simulink model "flightControlSystem"  (R2020a)
settings: Solver=ode3  StartTime=0  StopTime=TFinal  FixedStep=Ts  RelTol=1e-3  EnableMultiTasking=on
undefined symbols (not defined in the file): codertarget, Controller, DiscIntNeverNeededParam, Discrete, Estimator, g, gray, init, orient_ref, pos_ref, Sensors, Time, Ts, Vehicle
libraries: simulink x35, sharedtransform x3, ctrlSharedLib x2, sharedutil x1, visionstatistics x1, simulink_extras x1, parrotlib x1
(part 2 of 2)

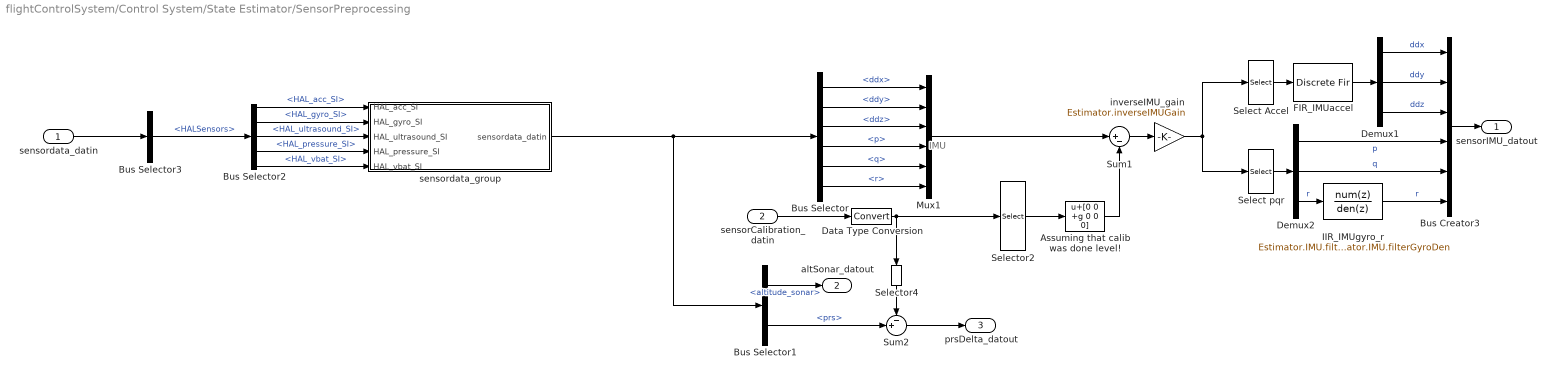
== system flightControlSystem/Control System/State Estimator/SensorPreprocessing ==
  note: IMU
  sensordata_datin : Inport
  sensorCalibration_datin : Inport  Port=2
  Assuming that calib was done level! : Bias  Bias=[0 0 +g 0 0 0]
  Bus Creator3 : BusCreator  Inputs=6
  Bus Selector : BusSelector  OutputSignals=ddx,ddy,ddz,p,q,r
  Bus Selector1 : BusSelector  OutputSignals=altitude_sonar,prs
  Bus Selector2 : BusSelector  OutputSignals=HAL_acc_SI,HAL_gyro_SI,HAL_ultrasound_SI,HAL_pressure_SI,HAL_vbat_SI
  Bus Selector3 : BusSelector  OutputSignals=HALSensors
  Data Type Conversion : DataTypeConversion
  Demux1 : Demux  Outputs=3
  Demux2 : Demux  Outputs=3
  FIR_IMUaccel : DiscreteFir  Coefficients=Estimator.IMU.filterAccel.Coefficients
  IIR_IMUgyro_r : DiscreteFilter  Numerator=Estimator.IMU.filterGyroNum  Denominator=Estimator.IMU.filterGyroDen
  Mux1 : Mux  Inputs=6
  Select Accel : Selector  InputPortWidth=6  IndexOptions=Index vector (dialog)  Indices=[1 2 3]  OutputSizes=1
  Select pqr : Selector  InputPortWidth=6  IndexOptions=Index vector (dialog)  Indices=[4 5 6]  OutputSizes=1
  Selector2 : Selector  InputPortWidth=8  IndexOptions=Index vector (dialog)  Indices=[1:6]  OutputSizes=1
  Selector4 : Selector  InputPortWidth=8  IndexOptions=Index vector (dialog)  Indices=[7]  OutputSizes=1
  Sum1 : Sum  Inputs=|+-
  Sum2 : Sum  Inputs=-+|
  inverseIMU_gain : Gain  Gain=Estimator.inverseIMUGain  ParamDataTypeStr=single  OutDataTypeStr=single
  sensordata_group : Subsystem
  sensorIMU_datout : Outport  VectorParamsAs1DForOutWhenUnconnected=off
  altSonar_datout : Outport  Port=2  VectorParamsAs1DForOutWhenUnconnected=off
  prsDelta_datout : Outport  Port=3  VectorParamsAs1DForOutWhenUnconnected=off
  wires:
  Select pqr/1 -> Demux2/1
  Assuming that calib was done level!/1 -> Sum1/2
  Mux1/1 -> Sum1/1
  Sum2/1 -> prsDelta_datout/1
  Bus Selector1/2 -> Sum2/2  "<prs>"
  Selector4/1 -> Sum2/1
  Bus Selector1/1 -> altSonar_datout/1  "<altitude_sonar>"
  Bus Selector/6 -> Mux1/6  "<r>"
  Bus Selector/5 -> Mux1/5  "<q>"
  Bus Selector/4 -> Mux1/4  "<p>"
  Bus Selector/3 -> Mux1/3  "<ddz>"
  Bus Selector/2 -> Mux1/2  "<ddy>"
  Bus Selector/1 -> Mux1/1  "<ddx>"
  sensorCalibration_datin/1 -> Data Type Conversion/1
  IIR_IMUgyro_r/1 -> Bus Creator3/6  "r"
  Demux2/3 -> IIR_IMUgyro_r/1  "r"
  FIR_IMUaccel/1 -> Demux1/1
  Select Accel/1 -> FIR_IMUaccel/1
  inverseIMU_gain/1 -> Select Accel/1, Select pqr/1
  Demux2/2 -> Bus Creator3/5  "q"
  Demux2/1 -> Bus Creator3/4  "p"
  Selector2/1 -> Assuming that calib was done level!/1
  Sum1/1 -> inverseIMU_gain/1
  Demux1/3 -> Bus Creator3/3  "ddz"
  Demux1/2 -> Bus Creator3/2  "ddy"
  Demux1/1 -> Bus Creator3/1  "ddx"
  Bus Creator3/1 -> sensorIMU_datout/1
  Data Type Conversion/1 -> Selector2/1, Selector4/1
  Bus Selector2/2 -> sensordata_group/2(HAL_gyro_SI)  "<HAL_gyro_SI>"
  Bus Selector2/4 -> sensordata_group/4(HAL_pressure_SI)  "<HAL_pressure_SI>"
  Bus Selector2/5 -> sensordata_group/5(HAL_vbat_SI)  "<HAL_vbat_SI>"
  Bus Selector2/3 -> sensordata_group/3(HAL_ultrasound_SI)  "<HAL_ultrasound_SI>"
  Bus Selector3/1 -> Bus Selector2/1  "<HALSensors>"
  sensordata_group/1(sensordata_datin) -> Bus Selector1/1, Bus Selector/1
  sensordata_datin/1 -> Bus Selector3/1
  Bus Selector2/1 -> sensordata_group/1(HAL_acc_SI)  "<HAL_acc_SI>"

== system flightControlSystem/Control System/Path Planning1/take current yaw, x and y targets in pixels, output the target orientation/create scaled x and y coordinates for finding an error angle less prone to fluctuation ==
  phi : Inport
  " y component in arbitrary coordinates" : Trigonometry
  scale y to reduce the angle : Gain  Gain=6
  x component in arbitrary coordinates : Trigonometry  Operator=cos
  x : Outport
  y : Outport  Port=2
  wires:
  phi/1 -> x component in arbitrary coordinates/1, " y component in arbitrary coordinates"/1
  scale y to reduce the angle/1 -> y/1
  " y component in arbitrary coordinates"/1 -> scale y to reduce the angle/1
  x component in arbitrary coordinates/1 -> x/1

== system flightControlSystem/Control System/Path Planning1/take current yaw, x and y targets in pixels, output the target orientation/output the desired yaw ==
  note: Subsystem
  note: Find the difference between absolute and relative angle
  note: relative angle, correction for 0 degrees at north (instead of east)
  note: Pump this through a logistic function so that smaller relative theta values are scaled less
  <yaw> : Inport
  a : Inport  Port=2
  Chart : Stateflow chart  TreatAsAtomicUnit=on
  Constant : Constant  Value=0
  Constant1 : Constant  Value=0
  Constant4 : Constant  Value=pi/2
  MATLAB Function : MATLAB Function  TreatAsAtomicUnit=on
  Minus2 : Sum  Inputs=+-
  Minus3 : Sum
  Scope : Scope
  z : Outport
  Out2 : Outport  Port=2
  Out3 : Outport  Port=3
  wires:
  Constant1/1 -> Out3/1
  Chart/1(z) -> z/1, Scope/1
  Minus3/1 -> Chart/1(input_theta)
  Constant4/1 -> Minus2/1
  Constant/1 -> Out2/1
  MATLAB Function/1(y) -> Minus3/2
  Minus2/1 -> MATLAB Function/1(u)
  a/1 -> Minus2/2
  <yaw>/1 -> Minus3/1

== system flightControlSystem/Control System/Path Planning1/take current yaw, x and y targets in pixels, output the target orientation/relative angle Phi of the pixel centre to the centre of mass measured anticlockwise from east in the frame of the drone ==
  note: angle in frame 1
  note: delX
  note: delY
  xcom : Inport
  ycom : Inport  Port=2
  Atan2 : Trigonometry  Operator=atan2
  Minus : Sum  Inputs=+-
  Minus1 : Sum  Inputs=+-
  x_pixel_grid_centre : Constant  Value=80
  y_pixel_grid_centre : Constant  Value=60
  Phi : Outport
  wires:
  xcom/1 -> Minus1/1
  y_pixel_grid_centre/1 -> Minus/1
  ycom/1 -> Minus/2
  Minus1/1 -> Atan2/2
  Minus/1 -> Atan2/1
  x_pixel_grid_centre/1 -> Minus1/2
  Atan2/1 -> Phi/1

== system flightControlSystem/Control System/Path Planning1/take current yaw, x and y targets in pixels, output the target orientation1/create scaled x and y coordinates for finding an error angle less prone to fluctuation ==
  phi : Inport
  " y component in arbitrary coordinates" : Trigonometry
  scale y to reduce the angle : Gain  Gain=2
  x component in arbitrary coordinates : Trigonometry  Operator=cos
  x : Outport
  y : Outport  Port=2
  wires:
  phi/1 -> x component in arbitrary coordinates/1, " y component in arbitrary coordinates"/1
  scale y to reduce the angle/1 -> y/1
  " y component in arbitrary coordinates"/1 -> scale y to reduce the angle/1
  x component in arbitrary coordinates/1 -> x/1

== system flightControlSystem/Control System/Path Planning1/take current yaw, x and y targets in pixels, output the target orientation1/output the desired yaw ==
  note: Subsystem
  note: Find the difference between absolute and relative angle
  note: relative angle, correction for 0 degrees at north (instead of east)
  note: Pump this through a logistic function so that smaller relative theta values are scaled less
  <yaw> : Inport
  a : Inport  Port=2
  Chart : Stateflow chart  TreatAsAtomicUnit=on
  Constant : Constant  Value=0
  Constant1 : Constant  Value=0
  Constant4 : Constant  Value=pi/2
  MATLAB Function : MATLAB Function  TreatAsAtomicUnit=on
  Minus2 : Sum  Inputs=+-
  Minus3 : Sum
  Scope : Scope
  z : Outport
  Out2 : Outport  Port=2
  Out3 : Outport  Port=3
  wires:
  Constant1/1 -> Out3/1
  Chart/1(z) -> z/1, Scope/1
  Minus3/1 -> Chart/1(input_theta)
  Constant4/1 -> Minus2/1
  Constant/1 -> Out2/1
  MATLAB Function/1(y) -> Minus3/2
  Minus2/1 -> MATLAB Function/1(u)
  a/1 -> Minus2/2
  <yaw>/1 -> Minus3/1

== system flightControlSystem/Control System/Path Planning1/take current yaw, x and y targets in pixels, output the target orientation1/relative angle Phi of the pixel centre to the centre of mass measured anticlockwise from east in the frame of the drone ==
  note: angle in frame 1
  note: delX
  note: delY
  xcom : Inport
  ycom : Inport  Port=2
  Atan2 : Trigonometry  Operator=atan2
  Minus : Sum  Inputs=+-
  Minus1 : Sum  Inputs=+-
  x_pixel_grid_centre : Constant  Value=80
  y_pixel_grid_centre : Constant  Value=60
  Phi : Outport
  wires:
  xcom/1 -> Minus1/1
  y_pixel_grid_centre/1 -> Minus/1
  ycom/1 -> Minus/2
  Minus1/1 -> Atan2/2
  Minus/1 -> Atan2/1
  x_pixel_grid_centre/1 -> Minus1/2
  Atan2/1 -> Phi/1

== system flightControlSystem/Control System/State Estimator/Complementary Filter/If Action Subsystem ==
  rpy : Inport
  accel : Inport  Port=2
  Action Port : ActionPort  ActionPortLabel=if(u1 > 0)
  Demux : Demux  Outputs=3
  Demux1 : Demux  Outputs=3
  Divide : Product  Inputs=*/
  Gain : Gain  Gain=1-Estimator.gyroAngleUpdateAccWeight
  Gain1 : Gain  Gain=Estimator.gyroAngleUpdateAccWeight
  Gain2 : Gain  Gain=1/g
  Gain3 : Gain  Gain=Estimator.gyroAngleUpdateAccWeight
  Gain4 : Gain  Gain=1-Estimator.gyroAngleUpdateAccWeight
  Mux : Mux  Inputs=2
  Sum : Sum  Inputs=|++
  Sum1 : Sum  Inputs=|++
  Terminator1 : Terminator
  Trigonometric Function : Trigonometry  Operator=atan
  Trigonometric Function1 : Trigonometry  Operator=asin
  pitch,roll : Outport  VectorParamsAs1DForOutWhenUnconnected=off
  wires:
  accel/1 -> Demux/1
  Demux/2 -> Divide/1
  Demux/3 -> Divide/2
  Divide/1 -> Trigonometric Function/1
  Gain/1 -> Sum/1
  Trigonometric Function/1 -> Gain1/1
  Mux/1 -> pitch,roll/1
  Gain2/1 -> Trigonometric Function1/1
  Trigonometric Function1/1 -> Gain3/1
  Gain4/1 -> Sum1/1
  Gain3/1 -> Sum1/2
  Sum1/1 -> Mux/1
  Sum/1 -> Mux/2
  rpy/1 -> Demux1/1
  Demux1/1 -> Gain/1
  Demux1/2 -> Gain4/1
  Demux/1 -> Gain2/1
  Demux1/3 -> Terminator1/1
  Gain1/1 -> Sum/2

== system flightControlSystem/Control System/State Estimator/Complementary Filter/If Action Subsystem2 ==
  prin : Inport
  Action Port : ActionPort  ActionPortLabel=else
  prout : Outport  VectorParamsAs1DForOutWhenUnconnected=off
  wires:
  prin/1 -> prout/1

== system flightControlSystem/Control System/State Estimator/Complementary Filter/Wbe ==
  rpy : Inport  OutDataTypeStr=single
  Constant : Constant  Value=single(0)
  Create 3x3 Matrix : sharedutil/Create 3x3 Matrix  aMode=aMode
      settings: SourceProductBaseCode=AE,PW,MT,VE,VP
  Divide : Product  Inputs=*/
  Gain : Gain  Gain=-1
  Product{1..4} (4 alike) : Product
  Selector : Selector  InputPortWidth=3  IndexOptions=Index vector (dialog)  Indices=[1]  OutputSizes=1
  Selector1 : Selector  InputPortWidth=3  IndexOptions=Index vector (dialog)  Indices=[1]  OutputSizes=1
  Selector2 : Selector  InputPortWidth=3  IndexOptions=Index vector (dialog)  Indices=[2]  OutputSizes=1
  Selector3 : Selector  InputPortWidth=3  IndexOptions=Index vector (dialog)  Indices=[2]  OutputSizes=1
  Trigonometric Function : Trigonometry  Operator=sincos
  Wbe : Outport  VectorParamsAs1DForOutWhenUnconnected=off
  wires:
  Create 3x3 Matrix/1 -> Divide/1
  Product3/1 -> Create 3x3 Matrix/8
  Trigonometric Function/2 -> Selector1/1, Selector2/1
  Selector3/1 -> Product4/2, Product3/2
  Selector1/1 -> Product4/1, Product1/1, Create 3x3 Matrix/3
  Trigonometric Function/1 -> Selector3/1, Selector/1
  Product1/1 -> Create 3x3 Matrix/5
  Product2/1 -> Create 3x3 Matrix/6
  Selector2/1 -> Divide/2, Create 3x3 Matrix/7, Product2/1, Product1/2
  Gain/1 -> Product2/2
  Product4/1 -> Create 3x3 Matrix/9
  Constant/1 -> Create 3x3 Matrix/4, Create 3x3 Matrix/1
  Divide/1 -> Wbe/1
  rpy/1 -> Trigonometric Function/1
  Selector/1 -> Product3/1, Gain/1, Create 3x3 Matrix/2

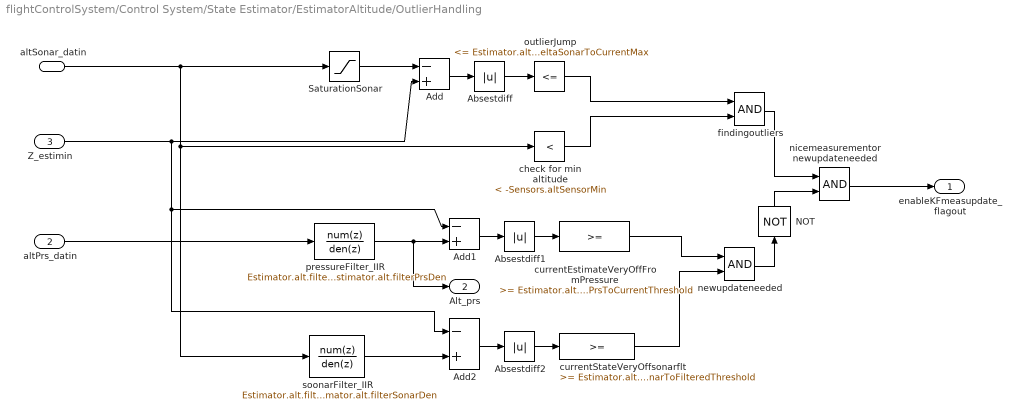
== system flightControlSystem/Control System/State Estimator/EstimatorAltitude/OutlierHandling ==
  altSonar_datin : Inport
  altPrs_datin : Inport  Port=2
  Z_estimin : Inport  Port=3
  Absestdiff : Abs
  Absestdiff1 : Abs
  Absestdiff2 : Abs
  Add : Sum  Inputs=-+
  Add1 : Sum  Inputs=-+
  Add2 : Sum  Inputs=-+
  NOT : Logic  Operator=NOT  IconShape=distinctive  AllPortsSameDT=off  OutDataTypeStr=boolean
  SaturationSonar : Saturate  UpperLimit=-Sensors.altSensorMin  LowerLimit=-inf
  check for min altitude : simulink/Logic and Bit Operations/Compare To Constant  relop=<  const=-Sensors.altSensorMin  OutDataTypeStr=boolean
  currentEstimateVeryOffFromPressure : simulink/Logic and Bit Operations/Compare To Constant  relop=>=  const=Estimator.alt.deltaPrsToCurrentThreshold  OutDataTypeStr=boolean
  currentStateVeryOffsonarflt : simulink/Logic and Bit Operations/Compare To Constant  relop=>=  const=Estimator.alt.deltaSonarToFilteredThreshold  OutDataTypeStr=boolean
  findingoutliers : Logic  AllPortsSameDT=off  OutDataTypeStr=boolean
  newupdateneeded : Logic  AllPortsSameDT=off  OutDataTypeStr=boolean
  nicemeasurementor newupdateneeded : Logic  AllPortsSameDT=off  OutDataTypeStr=boolean
  outlierJump : simulink/Logic and Bit Operations/Compare To Constant  relop=<=  const=Estimator.alt.deltaSonarToCurrentMax  OutDataTypeStr=boolean
  pressureFilter_IIR : DiscreteFilter  Numerator=Estimator.alt.filterPrsNum  Denominator=Estimator.alt.filterPrsDen
  soonarFilter_IIR : DiscreteFilter  Numerator=Estimator.alt.filterSonarNum  Denominator=Estimator.alt.filterSonarDen
  enableKFmeasupdate_flagout : Outport  VectorParamsAs1DForOutWhenUnconnected=off
  Alt_prs : Outport  Port=2  VectorParamsAs1DForOutWhenUnconnected=off
  wires:
  Add1/1 -> Absestdiff1/1
  nicemeasurementor newupdateneeded/1 -> enableKFmeasupdate_flagout/1
  findingoutliers/1 -> nicemeasurementor newupdateneeded/1
  check for min altitude/1 -> findingoutliers/2
  outlierJump/1 -> findingoutliers/1
  SaturationSonar/1 -> Add/1
  Absestdiff/1 -> outlierJump/1
  Add/1 -> Absestdiff/1
  newupdateneeded/1 -> NOT/1
  Absestdiff2/1 -> currentStateVeryOffsonarflt/1
  altSonar_datin/1 -> SaturationSonar/1, soonarFilter_IIR/1, check for min altitude/1
  currentEstimateVeryOffFromPressure/1 -> newupdateneeded/1
  Z_estimin/1 -> Add1/1, Add2/1, Add/2
  Add2/1 -> Absestdiff2/1
  currentStateVeryOffsonarflt/1 -> newupdateneeded/2
  pressureFilter_IIR/1 -> Alt_prs/1, Add1/2
  altPrs_datin/1 -> pressureFilter_IIR/1
  soonarFilter_IIR/1 -> Add2/2
  Absestdiff1/1 -> currentEstimateVeryOffFromPressure/1
  NOT/1 -> nicemeasurementor newupdateneeded/2

== system flightControlSystem/Control System/State Estimator/EstimatorXYPosition/EstimatorVelocity ==
  opticalFlow_datin : Inport
  Z_estimin : Inport  Port=2  SampleTime=Ts
  sensorIMU_datin : Inport  Port=3
  orient_estimin : Inport  Port=4
  " " : Product  Inputs=**
  AccelerationHandling : Subsystem
  Compare To Constant : simulink/Logic and Bit Operations/Compare To Constant  relop=<  const=200*4  OutDataTypeStr=boolean
  Counter Free-Running : simulink/Sources/Counter Free-Running  NumBits=32  tsamp=-1
  DataHandling : Subsystem
  Delay : Delay  DelayLength=1  InitialCondition=0
  Gain : Gain  Gain=-1
  KalmanFilter_dxdy : ctrlSharedLib/Kalman Filter  TimeDomain=Discrete-Time  UseCurrentEstimator=on  ModelSource=Individual A, B, C, D matrices  ModelSourceVariable=ss(0.95,1,1,0,1)  A=eye(2)  B=Ts*eye(2)  C=eye(2)  D=0  NumberOfStates=1  NumberOfInputs=1  NumberOfOutputs=1  InitialEstimateSource=Dialog  X0=0  P0=10  UseK=off  UseGH=on  NumberOfProcessNoiseInputs=1  G=Estimator.pos.kfVelo.G  TimeInvariantG=on  H=Estimator.pos.kfVelo.H  TimeInvariantH=on  Q=Estimator.pos.kfVelo.Q  TimeInvariantQ=on  R=Estimator.pos.kfVelo.R  TimeInvariantR=on  N=Estimator.pos.kfVelo.N  TimeInvariantN=on  AddInputPort=on  AddEnablePort=on  OutputEstimatedY=off  OutputP=off  Ts=-1
  Select dxy : Selector  InputPortWidth=3  IndexOptions=Index vector (dialog)  Indices=[1 2]  OutputSizes=1
  Switch : Switch  Criteria=u2 > Threshold
  Z_estimin1 : InportShadow  Port=2  SampleTime=Ts
  opticalFlowErrorCorrect : Gain  Gain=1.15
  dxy_estimout : Outport  VectorParamsAs1DForOutWhenUnconnected=off
  wires:
  Delay/1 -> DataHandling/5(dxyOF_datin)
  Z_estimin/1 -> DataHandling/1(Z_estimin), AccelerationHandling/4(Z_estimin)
  KalmanFilter_dxdy/1 -> dxy_estimout/1, Delay/1
  sensorIMU_datin/1 -> AccelerationHandling/2(sensorIMU_datin), DataHandling/3(sensorIMU_datin)
  orient_estimin/1 -> AccelerationHandling/3(orient_estimin), DataHandling/2(orient_estimin)
  Select dxy/1 -> KalmanFilter_dxdy/2, AccelerationHandling/1(dxy_estimin), DataHandling/4(dxy_estimin)
  AccelerationHandling/1(acceleration_world) -> KalmanFilter_dxdy/1
  DataHandling/1(enable_flag) -> KalmanFilter_dxdy/3
  Switch/1 -> Select dxy/1
  " "/1 -> opticalFlowErrorCorrect/1
  Gain/1 -> " "/2
  opticalFlowErrorCorrect/1 -> Switch/3
  Compare To Constant/1 -> Switch/2
  opticalFlow_datin/1 -> " "/1, Switch/1
  Z_estimin1/1 -> Gain/1
  Counter Free-Running/1 -> Compare To Constant/1

== system flightControlSystem/Control System/State Estimator/EstimatorXYPosition/EstimatorXYPosition ==
  note: Switching from orientationControl to Position
      | control reset the current world position estimate
      | (happens when using no markers)
  dxy_estimin : Inport
  orient_estimin : Inport  Port=2  SampleTime=Ts
  controlModePosVSOrient_flagin : Inport  Port=3
  dz_estimin : Inport  Port=4
  Math Function : Math  Operator=transpose  SignedPower=on  SaturateOnIntegerOverflow=on
  Mux2 : Mux  Inputs=2
  Product : Product  Multiplication=Matrix(*)
  Rotation Angles to Direction Cosine Matrix : sharedtransform/Rotation Angles to Direction Cosine Matrix  rotationOrder=ZYX  aMode=aMode
      settings: SourceProductBaseCode=AE,PW,MT,VE,VP
  SelectdXY : Selector  InputPortWidth=3  IndexOptions=Index vector (dialog)  Indices=[1 2]  OutputSizes=1
  SimplyIntegrateVelocity : DiscreteIntegrator  ExternalReset=rising  SampleTime=Ts  ICPrevOutput=DiscIntNeverNeededParam  ICPrevScaledInput=DiscIntNeverNeededParam
  XY_estimout : Outport  VectorParamsAs1DForOutWhenUnconnected=off
  wires:
  controlModePosVSOrient_flagin/1 -> SimplyIntegrateVelocity/2
  Product/1 -> SelectdXY/1
  Mux2/1 -> Product/2
  dz_estimin/1 -> Mux2/2
  SimplyIntegrateVelocity/1 -> XY_estimout/1
  dxy_estimin/1 -> Mux2/1
  orient_estimin/1 -> Rotation Angles to Direction Cosine Matrix/1
  Rotation Angles to Direction Cosine Matrix/1 -> Math Function/1
  SelectdXY/1 -> SimplyIntegrateVelocity/1
  Math Function/1 -> Product/1

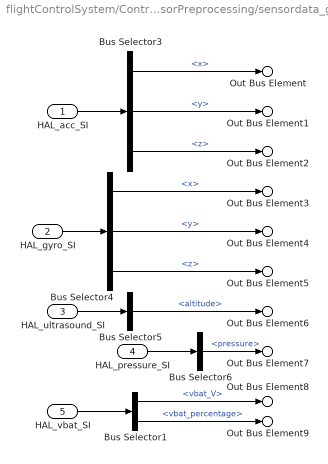
== system flightControlSystem/Control System/State Estimator/SensorPreprocessing/sensordata_group ==
  HAL_acc_SI : Inport  OutDataTypeStr=Bus: HAL_acc_SI_t
  HAL_gyro_SI : Inport  Port=2  OutDataTypeStr=Bus: HAL_gyro_SI_t
  HAL_ultrasound_SI : Inport  Port=3  OutDataTypeStr=Bus: HAL_ultrasound_SI_t
  HAL_pressure_SI : Inport  Port=4  OutDataTypeStr=Bus: HAL_pressure_SI_t
  HAL_vbat_SI : Inport  Port=5  OutDataTypeStr=Bus: HAL_vbat_SI_t
  Bus Selector1 : BusSelector  OutputSignals=vbat_V,vbat_percentage
  Bus Selector3 : BusSelector  OutputSignals=x,y,z
  Bus Selector4 : BusSelector  OutputSignals=x,y,z
  Bus Selector5 : BusSelector  OutputSignals=altitude
  Bus Selector6 : BusSelector  OutputSignals=pressure
  Out Bus Element : Outport  VectorParamsAs1DForOutWhenUnconnected=off  PortName=sensordata_datin  Element=ddx
  Out Bus Element1 : Outport  VectorParamsAs1DForOutWhenUnconnected=off  PortName=sensordata_datin  Element=ddy
  Out Bus Element2 : Outport  VectorParamsAs1DForOutWhenUnconnected=off  PortName=sensordata_datin  Element=ddz
  Out Bus Element3 : Outport  VectorParamsAs1DForOutWhenUnconnected=off  PortName=sensordata_datin  Element=p
  Out Bus Element4 : Outport  VectorParamsAs1DForOutWhenUnconnected=off  PortName=sensordata_datin  Element=q
  Out Bus Element5 : Outport  VectorParamsAs1DForOutWhenUnconnected=off  PortName=sensordata_datin  Element=r
  Out Bus Element6 : Outport  VectorParamsAs1DForOutWhenUnconnected=off  PortName=sensordata_datin  Element=altitude_sonar
  Out Bus Element7 : Outport  VectorParamsAs1DForOutWhenUnconnected=off  PortName=sensordata_datin  Element=prs
  Out Bus Element8 : Outport  VectorParamsAs1DForOutWhenUnconnected=off  PortName=sensordata_datin  Element=vbat_V
  Out Bus Element9 : Outport  VectorParamsAs1DForOutWhenUnconnected=off  PortName=sensordata_datin  Element=vbat_percentage
  wires:
  HAL_gyro_SI/1 -> Bus Selector4/1
  HAL_acc_SI/1 -> Bus Selector3/1
  HAL_pressure_SI/1 -> Bus Selector6/1
  HAL_ultrasound_SI/1 -> Bus Selector5/1
  Bus Selector4/1 -> Out Bus Element3/1  "<x>"
  Bus Selector3/3 -> Out Bus Element2/1  "<z>"
  Bus Selector4/3 -> Out Bus Element5/1  "<z>"
  Bus Selector5/1 -> Out Bus Element6/1  "<altitude>"
  Bus Selector6/1 -> Out Bus Element7/1  "<pressure>"
  Bus Selector4/2 -> Out Bus Element4/1  "<y>"
  Bus Selector3/1 -> Out Bus Element/1  "<x>"
  Bus Selector3/2 -> Out Bus Element1/1  "<y>"
  Bus Selector1/1 -> Out Bus Element8/1  "<vbat_V>"
  HAL_vbat_SI/1 -> Bus Selector1/1
  Bus Selector1/2 -> Out Bus Element9/1  "<vbat_percentage>"

== system flightControlSystem/Control System/State Estimator/EstimatorXYPosition/EstimatorVelocity/AccelerationHandling ==
  dxy_estimin : Inport
  sensorIMU_datin : Inport  Port=2
  orient_estimin : Inport  Port=3
  Z_estimin : Inport  Port=4
  Add : Sum  Inputs=-+
  Bus Selector1 : BusSelector  OutputSignals=ddx,ddy,ddz
  Deactivate Acceleration If OF is not used due to low altitude : simulink/Logic and Bit Operations/Compare To Constant  relop=<=  const=Estimator.pos.opticalFlowZMax  OutDataTypeStr=boolean
  Logical Operator : Logic  Operator=OR  AllPortsSameDT=off  OutDataTypeStr=boolean
  Mux6 : Mux  Inputs=3
  Product : Product  Inputs=3
  Product1 : Product  Multiplication=Matrix(*)
  Rotation Angles to Direction Cosine Matrix : sharedtransform/Rotation Angles to Direction Cosine Matrix  rotationOrder=ZYX  aMode=aMode
      settings: SourceProductBaseCode=AE,PW,MT,VE,VP
  SelectPlanarddxy : Selector  InputPortWidth=3  IndexOptions=Index vector (dialog)  Indices=[1 2]  OutputSizes=1
  Selector : Selector  InputPortWidth=2  IndexOptions=Index vector (dialog)  Indices=1  OutputSizes=1
  Selector1 : Selector  InputPortWidth=2  IndexOptions=Index vector (dialog)  Indices=2  OutputSizes=1
  do not use acc if optical flow never available (Note OF@60Hz but ZOH to 200!) : simulink/Logic and Bit Operations/Compare To Constant  relop=~=  const=0  OutDataTypeStr=boolean
  do not use acc if optical flow never available (Note OF@60Hz but ZOH to 200!)1 : simulink/Logic and Bit Operations/Compare To Constant  relop=~=  const=0  OutDataTypeStr=boolean
  gainaccinput : Gain  Gain=Estimator.pos.accelerationInputGain  OutDataTypeStr=single
  gravity : Constant  Value=[0 0 -g]
  acceleration_world : Outport  OutDataTypeStr=single  VectorParamsAs1DForOutWhenUnconnected=off
  wires:
  do not use acc if optical flow never available (Note OF@60Hz but ZOH to 200!)1/1 -> Logical Operator/2
  do not use acc if optical flow never available (Note OF@60Hz but ZOH to 200!)/1 -> Logical Operator/1
  Logical Operator/1 -> Product/1
  Selector1/1 -> do not use acc if optical flow never available (Note OF@60Hz but ZOH to 200!)1/1
  Selector/1 -> do not use acc if optical flow never available (Note OF@60Hz but ZOH to 200!)/1
  dxy_estimin/1 -> Selector1/1, Selector/1
  Product/1 -> acceleration_world/1
  Deactivate Acceleration If OF is not used due to low altitude/1 -> Product/3
  Z_estimin/1 -> Deactivate Acceleration If OF is not used due to low altitude/1
  Add/1 -> SelectPlanarddxy/1
  Product1/1 -> Add/1
  gravity/1 -> Product1/2
  gainaccinput/1 -> Product/2
  SelectPlanarddxy/1 -> gainaccinput/1
  Bus Selector1/3 -> Mux6/3  "<ddz>"
  Bus Selector1/1 -> Mux6/1  "<ddx>"
  sensorIMU_datin/1 -> Bus Selector1/1
  Mux6/1 -> Add/2
  Bus Selector1/2 -> Mux6/2  "<ddy>"
  orient_estimin/1 -> Rotation Angles to Direction Cosine Matrix/1
  Rotation Angles to Direction Cosine Matrix/1 -> Product1/1

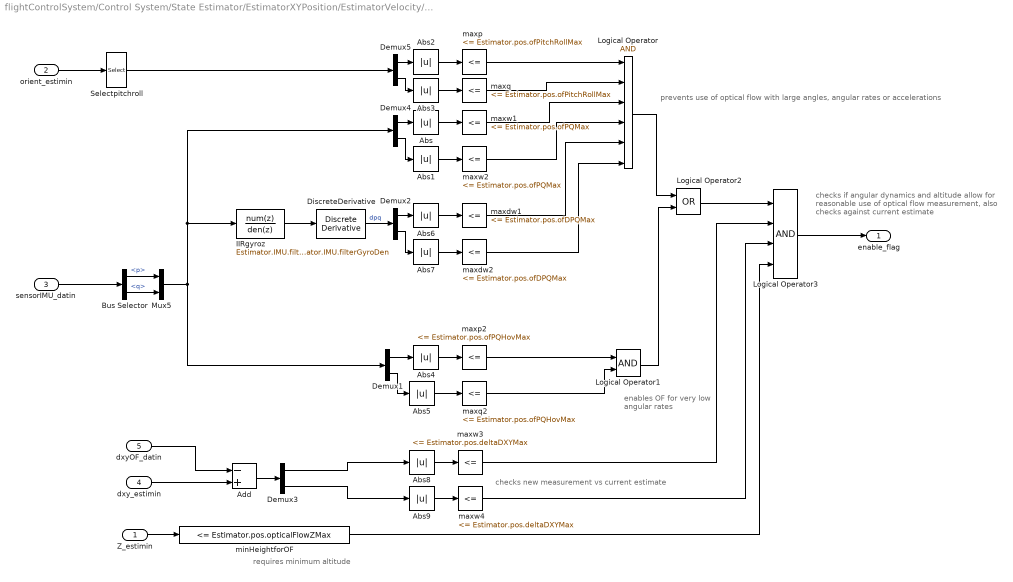
== system flightControlSystem/Control System/State Estimator/EstimatorXYPosition/EstimatorVelocity/DataHandling ==
  note: prevents use of optical flow with large angles, angular rates or accelerations
  note: enables OF for very
      | low angular rates
  note: checks if angular dynamics and altitude allow for
      | reasonable use of optical flow measurement,
      | also checks against current estimate
  note: checks new measurement vs current estimate
  note: requires minimum altitude
  Z_estimin : Inport
  orient_estimin : Inport  Port=2
  sensorIMU_datin : Inport  Port=3
  dxy_estimin : Inport  Port=4
  dxyOF_datin : Inport  Port=5
  Abs{,1..9} (10 alike) : Abs
  Add : Sum  Inputs=-+
  Bus Selector : BusSelector  OutputSignals=p,q
  Demux{1..5} (5 alike) : Demux  Outputs=2
  DiscreteDerivative : simulink/Discrete/Discrete Derivative  gainval=1.0  ICPrevScaledInput=0.0  OutMin=[]  OutMax=[]  OutDataType=fixdt(1, 16)  OutScaling=2^-10  DoSatur=off
  IIRgyroz : DiscreteFilter  Numerator=Estimator.IMU.filterGyroNum  Denominator=Estimator.IMU.filterGyroDen
  Logical Operator : Logic  Inputs=6  AllPortsSameDT=off  OutDataTypeStr=boolean
  Logical Operator1 : Logic  AllPortsSameDT=off  OutDataTypeStr=boolean
  Logical Operator2 : Logic  Operator=OR  AllPortsSameDT=off  OutDataTypeStr=boolean
  Logical Operator3 : Logic  Inputs=4  AllPortsSameDT=off  OutDataTypeStr=boolean
  Mux5 : Mux  Inputs=2
  Selectpitchroll : Selector  InputPortWidth=3  IndexOptions=Index vector (dialog)  Indices=[2 3]  OutputSizes=1
  maxdw1 : simulink/Logic and Bit Operations/Compare To Constant  relop=<=  const=Estimator.pos.ofDPQMax  OutDataTypeStr=boolean
  maxdw2 : simulink/Logic and Bit Operations/Compare To Constant  relop=<=  const=Estimator.pos.ofDPQMax  OutDataTypeStr=boolean
  maxp : simulink/Logic and Bit Operations/Compare To Constant  relop=<=  const=Estimator.pos.ofPitchRollMax  OutDataTypeStr=boolean
  maxp2 : simulink/Logic and Bit Operations/Compare To Constant  relop=<=  const=Estimator.pos.ofPQHovMax  OutDataTypeStr=boolean
  maxq : simulink/Logic and Bit Operations/Compare To Constant  relop=<=  const=Estimator.pos.ofPitchRollMax  OutDataTypeStr=boolean
  maxq2 : simulink/Logic and Bit Operations/Compare To Constant  relop=<=  const=Estimator.pos.ofPQHovMax  OutDataTypeStr=boolean
  maxw1 : simulink/Logic and Bit Operations/Compare To Constant  relop=<=  const=Estimator.pos.ofPQMax  OutDataTypeStr=boolean
  maxw2 : simulink/Logic and Bit Operations/Compare To Constant  relop=<=  const=Estimator.pos.ofPQMax  OutDataTypeStr=boolean
  maxw3 : simulink/Logic and Bit Operations/Compare To Constant  relop=<=  const=Estimator.pos.deltaDXYMax  OutDataTypeStr=boolean
  maxw4 : simulink/Logic and Bit Operations/Compare To Constant  relop=<=  const=Estimator.pos.deltaDXYMax  OutDataTypeStr=boolean
  minHeightforOF : simulink/Logic and Bit Operations/Compare To Constant  relop=<=  const=Estimator.pos.opticalFlowZMax  OutDataTypeStr=boolean
  enable_flag : Outport  VectorParamsAs1DForOutWhenUnconnected=off
  wires:
  minHeightforOF/1 -> Logical Operator3/4
  IIRgyroz/1 -> DiscreteDerivative/1
  Mux5/1 -> Demux1/1, IIRgyroz/1, Demux4/1
  maxw4/1 -> Logical Operator3/3
  maxw3/1 -> Logical Operator3/2
  dxyOF_datin/1 -> Add/1
  Demux3/2 -> Abs9/1
  Demux3/1 -> Abs8/1
  dxy_estimin/1 -> Add/2
  Add/1 -> Demux3/1
  Abs9/1 -> maxw4/1
  Abs8/1 -> maxw3/1
  Logical Operator2/1 -> Logical Operator3/1
  Logical Operator3/1 -> enable_flag/1
  DiscreteDerivative/1 -> Demux2/1  "dpq"
  Demux2/2 -> Abs7/1
  Demux2/1 -> Abs6/1
  Abs7/1 -> maxdw2/1
  Abs6/1 -> maxdw1/1
  Logical Operator1/1 -> Logical Operator2/2
  Demux1/2 -> Abs5/1
  Demux1/1 -> Abs4/1
  Abs5/1 -> maxq2/1
  Abs4/1 -> maxp2/1
  Abs3/1 -> maxq/1
  Abs2/1 -> maxp/1
  Demux4/2 -> Abs1/1
  Demux4/1 -> Abs/1
  Abs1/1 -> maxw2/1
  Abs/1 -> maxw1/1
  Z_estimin/1 -> minHeightforOF/1
  Logical Operator/1 -> Logical Operator2/1
  maxw1/1 -> Logical Operator/3
  Bus Selector/1 -> Mux5/1  "<p>"
  Selectpitchroll/1 -> Demux5/1
  sensorIMU_datin/1 -> Bus Selector/1
  maxq2/1 -> Logical Operator1/2
  Bus Selector/2 -> Mux5/2  "<q>"
  maxp/1 -> Logical Operator/1
  maxw2/1 -> Logical Operator/4
  orient_estimin/1 -> Selectpitchroll/1
  maxdw1/1 -> Logical Operator/5
  maxdw2/1 -> Logical Operator/6
  maxq/1 -> Logical Operator/2
  Demux5/1 -> Abs2/1
  Demux5/2 -> Abs3/1
  maxp2/1 -> Logical Operator1/1

== stateflow chart flightControlSystem/Control System/Path Planning1/take current yaw, x and y targets in pixels, output the target orientation1/output the desired yaw/Chart ==
  state Move1
    during:
    z=input_theta;
  state Takeoff
    entry:
    z=0;
  (default) -> Takeoff
  Takeoff -> Move1 : after(2, 'sec')
  data: z output; input_theta input

== matlab function flightControlSystem/Control System/Path Planning1/take current yaw, x and y targets in pixels, output the target orientation1/output the desired yaw/MATLAB Function ==
  data: u input; y output
function y = fcn(u)

y = u * (1/(1+ exp(-1-6*u)));
%y=u;

== matlab function flightControlSystem/Image Processing System/landing zone centre visualiser ==
  data: R_pix input; out output; LZ_x input; LZ_y input
function out = fcn(R_pix, LZ_x, LZ_y)

%if there are valid LZ_x and LZ_y values:
if ~isnan(LZ_x) && ~isnan(LZ_y) && (LZ_x > 3) && (LZ_y > 3)
    LZ_x = floor(LZ_x);
    xLo = LZ_x-2;
    xHi = LZ_x+2;

    LZ_y = floor(LZ_y);
    yLo = LZ_y-2;
    yHi = LZ_y+2;

    
    %Plot the centre of mass
    for i = (xLo):(xHi)
        for j = (yLo):(yHi)
            R_pix(j, i) = 0;
        end
    end
    
%     plot the centre of the viewing window
%     for i = (80-2):(80+2)
%        for j = (60-2):(60+2)
%            R_pix(j, i) = 0;
%        end
%     end

    out = R_pix;

else
    out = R_pix;
end


end

== matlab function flightControlSystem/Image Processing System/Landing zone detection flag and landing zone pixel centre/Colour_img_to_BW ==
  data: frame_info input size=[120, 160, 3]; y output size=[120, 160]
function y = fcn(frame_info)
% BW = [0, 0;
%       0, 0];
% coder.varsize('BW',[2, 2],[1, 1])
% coder.varsize('y',[120, 160, 3], [0, 0, 0])
% coder.varsize('u',[120, 160], [0, 0])
% coder.varsize('statsOneObj.PixelIdxList',[1000000 1],[1 0]);

% stats = regionprops(u, 'Area')



% Convert RGB image to chosen color space
I = rgb2hsv(frame_info);


% Define thresholds for channel 1 based on histogram settings
channel1Min = 0.938;
channel1Max = 0.000;

% Define thresholds for channel 2 based on histogram settings
channel2Min = 0.419;
channel2Max = 1.000;

% Define thresholds for channel 3 based on histogram settings
channel3Min = 0.841;
channel3Max = 1.000;

% Create mask based on chosen histogram thresholds
sliderBW = ( (I(:,:,1) >= channel1Min) | (I(:,:,1) <= channel1Max) ) & ...
    (I(:,:,2) >= channel2Min ) & (I(:,:,2) <= channel2Max) & ...
    (I(:,:,3) >= channel3Min ) & (I(:,:,3) <= channel3Max);
% BW = (zeros(2, 2));
BW = sliderBW;
y = BW;

% 
% stats = regionprops(BW, 'Area')
% 
% threshold = 0.94;

% y = u;

== matlab function flightControlSystem/Image Processing System/Landing zone detection flag and landing zone pixel centre/MATLAB Function1 ==
  data: eccentricity input; Lz_flag output; Lz_x output; Lz_y output; area input; centre input
function [Lz_flag, Lz_x, Lz_y] = fcn(eccentricity, area, centre)

%values for when the landing zone has not been sighted
Lz_flag = logical(0);
%these are not acted on
Lz_x = 80;
Lz_y = 60;

%eccentricity threshold for detecting a circle
threshold = 0.25;


e_size = size(eccentricity);
for i=1:50
    
    if eccentricity(i) < threshold && eccentricity(i) > 0.01
        if area(i) > 0
            if area(i) < 100000000
                Lz_flag = logical(1);
                Lz_x = centre(i, 1);
                Lz_y = centre(i, 2);
            end
        end
    end
end

== matlab function flightControlSystem/Image Processing System/LZ_flag is set to 1 when the landing zone is detected, and 0 otherwise ==
  data: frame_info input; LZ_flag output; LZ_x output; LZ_y output
function [LZ_flag, LZ_x, LZ_y] = fcn(frame_info)


%% Load sample frames
% subplot(3, 1, 1);
% imshow(frame);

%% Video thresholding
% Convert RGB image to chosen color space
I = rgb2hsv(frame_info);

% Define thresholds for channel 1 based on histogram settings
channel1Min = 0.986;
channel1Max = 0.026;

% Define thresholds for channel 2 based on histogram settings
channel2Min = 0.000;
channel2Max = 1.000;

% Define thresholds for channel 3 based on histogram settings
channel3Min = 0.906;
channel3Max = 1.000;

% Create mask based on chosen histogram thresholds
sliderBW = ( (I(:,:,1) >= channel1Min) | (I(:,:,1) <= channel1Max) ) & ...
    (I(:,:,2) >= channel2Min ) & (I(:,:,2) <= channel2Max) & ...
    (I(:,:,3) >= channel3Min ) & (I(:,:,3) <= channel3Max);
BW = sliderBW;



%% Get rid of image fuzz

%% Analysis using circularity





%% Blob analysis
hBlobAnalysis = vision.BlobAnalysis('MinimumBlobArea', 1, 'MaximumBlobArea', 100000);
[objectArea, objCentroid, bboxOut] = step(hBlobAnalysis, BW);

size_of_bbox = size(bboxOut);
%allowable error (in pixels)
err = 10;
squareness_threshold = 15;

%start by assuming we aren't near the landing zone
LZ_flag = int32(0);
LZ_x = int32(0);
LZ_y = int32(0);

for i=1:size_of_bbox(1)
    
    % Tests for the blob being square enough and the right size to be the
    % landing zone (LZ)
           %width              %height
    if (abs(bboxOut(i, 3) - bboxOut(i, 4)) < squareness_threshold)...
            && ((bboxOut(i, 3) > 42-err) && (bboxOut(i, 3) < 42 + err))
            %detected landing zone
            LZ_flag = int32(1);       
            %the coordinates describing the centre of the landing zone
            %PURPOSELY REVERSED SO THAT THEY ARE IN THE SAME FORMAT 
            % AS XCOM,YCOM, IE X IS LEFT/RIGHT AND Y IS UP/DOWN
            LZ_x = bboxOut(i, 1) + bboxOut(i, 3)/2; %might be + height/2 instead THIS ERROR WOULD BE HARD TO DETECT
            LZ_y = bboxOut(i, 2) + bboxOut(i, 4)/2; 
    end
end


%% Annotate the image
% Ishape = insertShape(frame_info, 'rectangle', bboxOut, 'Linewidth', 5);
% y = Ishape;

== matlab function flightControlSystem/Image Processing System/find the weighted path centre ==
  data: R_pixels input; G_pixels input; xcom output; B_pixels input; ycom output
% Image Processing System:
% goal: find the CoM of the red pixels
% 
% Notes:
% -need to know where the pixel array starts. is (1,1) the top left?



% compute the weighted centroid of the pixels on the screen belonging to the path
% arguments: R_pixels is the array of the R values for each pixel, etc
function [xcom,ycom] = find_path_centre(R_pixels, G_pixels, B_pixels)

    NUM_ROWS = 120;
    NUM_COLS = 160;
    
    %These need to be updated
    THRESHOLD = 180;
    BOTTOM_ROW_INDEX = 120;
    TOP_ROW_INDEX = 1;
    
    %preallocate two weights arrays
    %this array weights the rows
    vertical_weights = zeros(160);
    %this array weights the columns
    horizontal_weights = zeros(160);
    
    %initially paint all pixels as being off the path (maybe remove?)
    for row = 1:NUM_ROWS
		for col = 1:NUM_COLS
            vertical_weights(row,col) = 0;
            horizontal_weights(row,col) = 0;
        end
    end
    
    %define the restricted view window
    d_pix = 50;
    MIN_ROW = NUM_ROWS/2 - d_pix/2;%for entire window: 1
    MAX_ROW = NUM_ROWS/2 + d_pix/2;%                   NUM_ROWS
    MIN_COL = NUM_COLS/2 - 1.3*d_pix;%                   1
    MAX_COL = NUM_COLS/2 + 1.3*d_pix;%                   NUM_COLS
    
	%For all pixels within the restricted view window
	for row = MIN_ROW:MAX_ROW
		for col = MIN_COL:MAX_COL

% 			%Evaluate against redness threshold:		
% 			%if the pixel is deemed 'red' set its weight based on how far in front or behind the drone it is:
			if (R_pixels(row,col) > THRESHOLD)

                %weighting scales from MIN_WEIGHT (the bottom row of pixels) to MAX_WEIGHT (the top row of pixels)
                MIN_WEIGHT = 0;%0
                MAX_WEIGHT = 4;%100
                
                %only consider top X% of pixels
                %if row < 2*NUM_ROWS/10
                if row < (MIN_ROW + 4*(MAX_ROW - MIN_ROW)/10)    
                weight = MIN_WEIGHT + ((MIN_ROW - row) / (MIN_ROW - MAX_ROW)) * (MAX_WEIGHT - MIN_WEIGHT);
                    vertical_weights(row,col) = weight;
                else
                    vertical_weights(row,col)=0;
                end
                                 
%               weight = MIN_WEIGHT + (BOTTOM_ROW_INDEX - row) / (BOTTOM_ROW_INDEX - TOP_ROW_INDEX) * (MAX_WEIGHT - MIN_WEIGHT);
%               vertical_weights(row,col) = weight;            
                
                %for purposes of determining the horizontal CoM component, all
                %points on the path have weight 1
                horizontal_weights(row,col) = 1;
               
                %OR give further points from the centre higher weight
%                 horizontal_weights(row,col) = MIN_WEIGHT + (abs(MAX_COL/2 - col) / (MIN_COL - MAX_COL)) * (MAX_WEIGHT - MIN_WEIGHT);
%               
%             
% 			%if the pixel is not deemed a part of the path, set its weight to 0
			else 
				vertical_weights(row,col) = 0;
                horizontal_weights(row,col) = 0;
            end
        end
    end
%     
% 	
% 	%Compute the centre of mass of the pixels (regular CoM formula where the mass is instead the pixel weight)
% 	
% 	%find the centre of mass x and y coordinate (round down because pixel positions have integer designations)
	xcom_numerator = 0;
    xcom_denominator = 0;
    ycom_numerator = 0;
    ycom_denominator = 0;
	
	for row = 1:NUM_ROWS
		for col = 1:NUM_COLS
			xcom_numerator = xcom_numerator + row * vertical_weights(row,col);
			xcom_denominator = xcom_denominator + vertical_weights(row,col);
			ycom_numerator = ycom_numerator + col * horizontal_weights(row,col);
			ycom_denominator = ycom_denominator + horizontal_weights(row,col);
%             ycom_numerator = ycom_numerator + col * vertical_weights(row,col);
% 			ycom_denominator = ycom_denominator + vertical_weights(row,col);
        end
    end

	%compute coordinates of centre of mass
    % xcom and ycom are reversed because x and y are left/right and up/down
    % respectively
    %additional protections for no path pixels being seen 
    if xcom_denominator == 0
        ycom = 10;
    else
        ycom = floor(xcom_numerator / xcom_denominator);
    end
    
    if ycom_denominator == 0        
        xcom = 10;
    else 
        xcom = floor(ycom_numerator / ycom_denominator);
    end
    


end

== stateflow chart flightControlSystem/Control System/Path Planning1/take current yaw, x and y targets in pixels, output the target orientation/output the desired yaw/Chart ==
  state Move1
    during:
    z=input_theta;
  state Takeoff
    entry:
    z=0;
  (default) -> Takeoff
  Takeoff -> Move1 : after(2, 'sec')
  data: z output; input_theta input

== stateflow chart flightControlSystem/Control System/Path Planning1/position_states ==
  state Start
    entry:
    x_out=0;
    y_out=0;
    z_out=-1;
  state Step1
    during:
    speed_factor = 2200;
    x_out= x_out + cos(theta)/speed_factor;
    y_out=y_out + sin(theta)/speed_factor;
  (default) -> Start
  Start -> Step1 : after(6,'sec')
  data: x_in input; y_in input; z_in input; x_out output; y_out output; z_out output; theta input; speed_factor local; x_nudge input

== matlab function flightControlSystem/Image Processing System/path centre visualiser ==
  data: R_pix input; out output; xcom input; ycom input
function out = fcn(R_pix, xcom, ycom)

%if there are valid xcom and ycom values:
if ~isnan(xcom) && ~isnan(ycom) && xcom > 4 && ycom > 4
    xcom = floor(xcom);
    xLo = xcom-4;
    xHi = xcom+4;

    ycom = floor(ycom);
    yLo = ycom-4;
    yHi = ycom+4;

    
    %Plot the centre of mass
    for i = (xLo):(xHi)
        for j = (yLo):(yHi)
            R_pix(j, i) = 0;
        end
    end
    
    for i = (80-4):(80+4)
        for j = (60-4):(60+4)
            R_pix(j, i) = 0;
        end
    end

    out = R_pix;

else
    out = R_pix;
end


end

== matlab function flightControlSystem/Control System/Path Planning1/take current yaw, x and y targets in pixels, output the target orientation/output the desired yaw/MATLAB Function ==
  data: u input; y output
function y = fcn(u)

y = u * (1/(1+ exp(-1-6*u)));
%y=u;

== stateflow chart flightControlSystem/Control System/Path Planning1/Determine which reference signals to pass based on the flight stage ==
  state Path_Following
    during:
    ref_out = path_following_ref;
  state Landing
    during:
    ref_out = landing_ref;
  (default) -> Path_Following
  Path_Following -> Landing : [LZ_flag > 0.5 ]
  data: LZ_flag input; path_following_ref input; landing_ref input; ref_out output

== matlab function flightControlSystem/Control System/Path Planning1/Position states during landing ==
  data: target_yaw input; x output; LZ_x input; y output; LZ_y input; z output; current_x input; current_y input; current_z input; locked_on output
function [x,y,z,locked_on] = new_landing_states(target_yaw, LZ_x, LZ_y, current_x, current_y, current_z)
%NOTE: CHECK THESE ARE THE CORRECT WAY AROUND
X_PIXEL_GRID_CENTRE = 80;
Y_PIXEL_GRID_CENTRE = 60;

%indicate if close enough to the landing zone centre
locked_on = (abs(LZ_x - X_PIXEL_GRID_CENTRE) < 10) && (abs(LZ_y - Y_PIXEL_GRID_CENTRE) < 10);
    
%if not close enough to the landing zone centre, progress towards it
%this should use similar logic to the angle calculations 
if ~locked_on
    x = current_x + cos(target_yaw)/900;
    y = current_y + sin(target_yaw)/900;
    z = current_z; %should be z = previous_zref

%if close enough to the LZ centre, land
else
    %hold x and y constant
    x = current_x; %want x_ref = previous x_ref
    y = current_y; %
    
    %decrement z, or turn off the drone when z is low enough
    if abs(current_z) < 0.1
        z = current_z;  %want z_ref = previous z_ref   
    else
        z = current_z + 0.1; % want z_ref = previous z_ref + 0.1
    end
end
